simulink model "snap2_f_200msps_64i_4096c"  (R2019a)
settings: Solver=VariableStepDiscrete  StartTime=0.0  StopTime=10.0  RelTol=1e-3
undefined symbols (not defined in the file or in its folder): datetime, posixtime
libraries: xbsIndex_r4 x21354, casper_library_misc x297, casper_library_delays x19, xps_library x14, casper_library_sources x4
(part 9 of 217)

== system snap2_f_200msps_64i_4096c/autocorr/0 ==
  note: new_acc should precede data by a cycle
  note: acc length in spectra
  note: clock after sync counter goes to 1.
      |
      | Equality test goes high N spectra clock after sync. I.e., goes high with the last sample of the last spectra
  note: starts on 1
  sync : Inport
  din : Inport  Port=2
  rst : Inport  Port=3
  acc_len : Inport  Port=4
  trig : Inport  Port=5
  Convert{,1..7} (8 alike) : xbsIndex_r4/Convert  gui_display_data_type=Floating-point  arith_type=Floating-point  n_bits=16  bin_pt=14  float_type=Single  exp_bits=8  fraction_bits=24  quantization=Truncate  overflow=Wrap  en=off  latency=4  pipeline=on  dbl_ovrd=off  block_type=convert
  Counter : xbsIndex_r4/Counter  cnt_type=Free Running  cnt_to=Inf  operation=Up  start_count=1  cnt_by_val=1  arith_type=Unsigned  n_bits=30  bin_pt=0  load_pin=off  rst=on  en=off  explicit_period=on  period=1  use_behavioral_HDL=off  implementation=Fabric  dbl_ovrd=off  block_type=counter
  Delay : xbsIndex_r4/Delay  rst=off  infoeditControl=Selection of Reset will increase slice count due to use of real FFs and instead of SRLs  en=off  latency=1  reg_retiming=off  dbl_ovrd=off  block_type=delay
  Delay{1..16} (16 alike) : xbsIndex_r4/Delay  rst=off  infoeditControl=Selection of Reset will increase slice count due to use of real FFs and instead of SRLs  en=off  latency=4  reg_retiming=off  dbl_ovrd=off  block_type=delay
  Delay{17..32} (16 alike) : xbsIndex_r4/Delay  rst=off  infoeditControl=Selection of Reset will increase slice count due to use of real FFs and instead of SRLs  en=off  latency=1  reg_retiming=on  dbl_ovrd=off  block_type=delay
  Logical : xbsIndex_r4/Logical  logical_function=OR  inputs=2  en=off  latency=0  precision=Full  arith_type=Unsigned  n_bits=16  bin_pt=0  align_bp=on  dbl_ovrd=off  block_type=logical
  Logical{1..9} (9 alike) : xbsIndex_r4/Logical  logical_function=AND  inputs=2  en=off  latency=0  precision=Full  arith_type=Unsigned  n_bits=16  bin_pt=0  align_bp=on  dbl_ovrd=off  block_type=logical
  Register1 : xbsIndex_r4/Register  init=0  rst=on  en=on  dbl_ovrd=off  block_type=register
  Reinterpret{,1..7} (8 alike) : xbsIndex_r4/Reinterpret  force_arith_type=on  arith_type=Unsigned  force_bin_pt=on  bin_pt=0  block_type=reinterpret
  Relational : xbsIndex_r4/Relational  mode=a=b  op_type=Bool  en=off  latency=0  dbl_ovrd=off  block_type=relational
  Slice : xbsIndex_r4/Slice  nbits=30-nchan_bits-npol_bits  boolean_output=off  mode=Lower Bit Location + Width  bit1=0  base1=MSB of Input  bit0=nchan_bits + npol_bits  base0=LSB of Input  dbl_ovrd=off  block_type=slice
  bus_expand : Subsystem  AncestorBlock=casper_library_flow_control/bus_expand  mask(bus_expand){mode=divisions of equal size, outputNum=8, outputWidth=36, outputBinaryPt=0, outputArithmeticType=0, show_format=off, outputToWorkspace=off, variablePrefix=out, outputToModelAsWell=on}
      mask prompts: outputNum "Number of outputs:"; outputWidth "Output width:"; outputBinaryPt "Output binary point position:"; outputArithmeticType "Output arithmetic type (ufix=0, fix=1, bool=2):"; show_format "Print format string?"; outputToWorkspace "Output to workspace?"; variablePrefix "Variable name prefix:"; outputToModelAsWell "Output to model as well?"
      mask help:
      | Expands a 'bus' made using a bus_create or Xilinx
      | concat block.
      | The input will be divided into the specified number
      | of outputs with the specified arithmetic types.
      | Divisions are made from most significant bit.
      mask init: same as snap2_f_200msps_64i_4096c/autocorr/bus_expand
      settings: AttributesFormatString=8 outputs
      mask TypeOptions mode: divisions of equal size | divisions of arbitrary size
      mask Callback mode: bus_expand_callback();
      mask Callback outputWidth: bus_expand_callback();
      mask Callback outputToWorkspace: bus_expand_callback();
  dout0 : Subsystem
  dout1 : Subsystem
  dout2 : Subsystem
  dout3 : Subsystem
  dout4 : Subsystem
  dout5 : Subsystem
  dout6 : Subsystem
  dout7 : Subsystem
  edge_detect{,1..2,4} (4 alike) : casper_library_misc/edge_detect  edge=Rising  polarity=Active High  x_in=[0 0.08 0.08 0.16 0.16 0.24 0.24 0.32 0.32 0.4]  y_in="[-1 -1  1  1  1  1  1  1  1  1]"  x_out=[0.6 0.68 0.68 0.76 0.76 0.84 0.84 0.92 0.92 1]  y_out="[-1 -1  1  1 -1 -1 -1 -1 -1 -1]"
  edge_detect3 : Subsystem  AncestorBlock=casper_library_misc/edge_detect  mask(edge_detect){edge=Falling, polarity=Active High, x_in=[0 0.08 0.08 0.16 0.16 0.24 0.24 0.32 0.32 0.4], y_in=[-1 -1  1  1  1  1  1  1  1  1], x_out=[0.6 0.68 0.68 0.76 0.76 0.84 0.84 0.92 0.92 1], y_out=[-1 -1  1  1 -1 -1 -1 -1 -1 -1]}
      mask prompts: edge "Edge Type"; polarity "Output Polarity"; x_in "Input X Positions"; y_in "Input Y Positions"; x_out "Output X Positions"; y_out "Output Y Positions"
      mask help: Output is active for one-cycle after each edge of the specified type (i.e. rising, falling or both).
      mask init: same as snap2_f_200msps_64i_4096c/cosmic_ray/edge_detect
      settings: AttributesFormatString=|
      | falling edges
      | active high
      mask Help: Output is active for one-cycle after each edge of the specified type (i.e. rising, falling, or both).  Latency is zero.
      mask TypeOptions edge: Rising | Falling | Both
      mask TypeOptions polarity: Active High | Active Low
      mask Display:
      | plot(x_in_num,0.5+y_in_num*0.2);
      | plot(x_out_num,0.5+y_out_num*0.2);
  en_reg : xbsIndex_r4/Register  init=0  rst=on  en=on  dbl_ovrd=off  block_type=register
  power_dsp48e{,1..7} (8 alike) : casper_library_misc/power_dsp48e  bitwidth=18
      settings: SourceProductName=CASPER DSP Blockset
  simple_bram_vacc0 : Subsystem  AncestorBlock=casper_library_accumulators/simple_bram_vacc  mask(simple_bram_vacc){vec_len=2^(nchan_bits + npol_bits), arith_type=Signed, n_bits=64, bin_pt=17*2}
      mask prompts: vec_len "Vector length:"; arith_type "Output type:"; n_bits "Bit width (output):"; bin_pt "Binary point (output):"
      mask help: This simple vector accumulator is based on a shift register. It outputs its previous accumulated vector after a new_acc pulse is received.
      mask init:
      | simple_bram_vacc_init(gcb, ...
      |     'vec_len', vec_len, ...
      |     'arith_type', arith_type, ...
      |     'n_bits', n_bits, ...
      |     'bin_pt', bin_pt);
      mask TypeOptions arith_type: Signed | Unsigned
  simple_bram_vacc1 : Subsystem  AncestorBlock=casper_library_accumulators/simple_bram_vacc  mask(simple_bram_vacc){vec_len=2^(nchan_bits + npol_bits), arith_type=Signed, n_bits=64, bin_pt=17*2}
      mask prompts: vec_len "Vector length:"; arith_type "Output type:"; n_bits "Bit width (output):"; bin_pt "Binary point (output):"
      mask help: This simple vector accumulator is based on a shift register. It outputs its previous accumulated vector after a new_acc pulse is received.
      mask init:
      | simple_bram_vacc_init(gcb, ...
      |     'vec_len', vec_len, ...
      |     'arith_type', arith_type, ...
      |     'n_bits', n_bits, ...
      |     'bin_pt', bin_pt);
      mask TypeOptions arith_type: Signed | Unsigned
  simple_bram_vacc2 : Subsystem  AncestorBlock=casper_library_accumulators/simple_bram_vacc  mask(simple_bram_vacc){vec_len=2^(nchan_bits + npol_bits), arith_type=Signed, n_bits=64, bin_pt=17*2}
      mask prompts: vec_len "Vector length:"; arith_type "Output type:"; n_bits "Bit width (output):"; bin_pt "Binary point (output):"
      mask help: This simple vector accumulator is based on a shift register. It outputs its previous accumulated vector after a new_acc pulse is received.
      mask init:
      | simple_bram_vacc_init(gcb, ...
      |     'vec_len', vec_len, ...
      |     'arith_type', arith_type, ...
      |     'n_bits', n_bits, ...
      |     'bin_pt', bin_pt);
      mask TypeOptions arith_type: Signed | Unsigned
  simple_bram_vacc3 : Subsystem  AncestorBlock=casper_library_accumulators/simple_bram_vacc  mask(simple_bram_vacc){vec_len=2^(nchan_bits + npol_bits), arith_type=Signed, n_bits=64, bin_pt=17*2}
      mask prompts: vec_len "Vector length:"; arith_type "Output type:"; n_bits "Bit width (output):"; bin_pt "Binary point (output):"
      mask help: This simple vector accumulator is based on a shift register. It outputs its previous accumulated vector after a new_acc pulse is received.
      mask init:
      | simple_bram_vacc_init(gcb, ...
      |     'vec_len', vec_len, ...
      |     'arith_type', arith_type, ...
      |     'n_bits', n_bits, ...
      |     'bin_pt', bin_pt);
      mask TypeOptions arith_type: Signed | Unsigned
  simple_bram_vacc4 : Subsystem  AncestorBlock=casper_library_accumulators/simple_bram_vacc  mask(simple_bram_vacc){vec_len=2^(nchan_bits + npol_bits), arith_type=Signed, n_bits=64, bin_pt=17*2}
      mask prompts: vec_len "Vector length:"; arith_type "Output type:"; n_bits "Bit width (output):"; bin_pt "Binary point (output):"
      mask help: This simple vector accumulator is based on a shift register. It outputs its previous accumulated vector after a new_acc pulse is received.
      mask init:
      | simple_bram_vacc_init(gcb, ...
      |     'vec_len', vec_len, ...
      |     'arith_type', arith_type, ...
      |     'n_bits', n_bits, ...
      |     'bin_pt', bin_pt);
      mask TypeOptions arith_type: Signed | Unsigned
  simple_bram_vacc5 : Subsystem  AncestorBlock=casper_library_accumulators/simple_bram_vacc  mask(simple_bram_vacc){vec_len=2^(nchan_bits + npol_bits), arith_type=Signed, n_bits=64, bin_pt=17*2}
      mask prompts: vec_len "Vector length:"; arith_type "Output type:"; n_bits "Bit width (output):"; bin_pt "Binary point (output):"
      mask help: This simple vector accumulator is based on a shift register. It outputs its previous accumulated vector after a new_acc pulse is received.
      mask init:
      | simple_bram_vacc_init(gcb, ...
      |     'vec_len', vec_len, ...
      |     'arith_type', arith_type, ...
      |     'n_bits', n_bits, ...
      |     'bin_pt', bin_pt);
      mask TypeOptions arith_type: Signed | Unsigned
  simple_bram_vacc6 : Subsystem  AncestorBlock=casper_library_accumulators/simple_bram_vacc  mask(simple_bram_vacc){vec_len=2^(nchan_bits + npol_bits), arith_type=Signed, n_bits=64, bin_pt=17*2}
      mask prompts: vec_len "Vector length:"; arith_type "Output type:"; n_bits "Bit width (output):"; bin_pt "Binary point (output):"
      mask help: This simple vector accumulator is based on a shift register. It outputs its previous accumulated vector after a new_acc pulse is received.
      mask init:
      | simple_bram_vacc_init(gcb, ...
      |     'vec_len', vec_len, ...
      |     'arith_type', arith_type, ...
      |     'n_bits', n_bits, ...
      |     'bin_pt', bin_pt);
      mask TypeOptions arith_type: Signed | Unsigned
  simple_bram_vacc7 : Subsystem  AncestorBlock=casper_library_accumulators/simple_bram_vacc  mask(simple_bram_vacc){vec_len=2^(nchan_bits + npol_bits), arith_type=Signed, n_bits=64, bin_pt=17*2}
      mask prompts: vec_len "Vector length:"; arith_type "Output type:"; n_bits "Bit width (output):"; bin_pt "Binary point (output):"
      mask help: This simple vector accumulator is based on a shift register. It outputs its previous accumulated vector after a new_acc pulse is received.
      mask init:
      | simple_bram_vacc_init(gcb, ...
      |     'vec_len', vec_len, ...
      |     'arith_type', arith_type, ...
      |     'n_bits', n_bits, ...
      |     'bin_pt', bin_pt);
      mask TypeOptions arith_type: Signed | Unsigned
  trig_reg : xbsIndex_r4/Register  init=0  rst=on  en=on  dbl_ovrd=off  block_type=register
  new_acc : Outport
  wires:
  trig/1 -> edge_detect2/1
  Delay32/1 -> Logical9/1
  Delay31/1 -> Logical8/1
  Delay30/1 -> Logical7/1
  Delay29/1 -> Logical6/1
  Delay28/1 -> Logical5/1
  Delay27/1 -> Logical4/1
  Delay26/1 -> Logical3/1
  Delay14/1 -> Delay30/1
  Delay13/1 -> Delay29/1
  Delay12/1 -> Delay28/1
  Delay11/1 -> Delay27/1
  Delay10/1 -> Delay26/1
  Delay25/1 -> Logical1/1
  Delay15/1 -> Delay31/1
  Delay16/1 -> Delay32/1
  Logical9/1 -> dout7/2(vld)
  Logical8/1 -> dout6/2(vld)
  Logical7/1 -> dout5/2(vld)
  Logical6/1 -> dout4/2(vld)
  Logical5/1 -> dout3/2(vld)
  [enable_write] -> Logical9/2
  [enable_write] -> Logical8/2
  [enable_write] -> Logical7/2
  [enable_write] -> Logical6/2
  [enable_write] -> Logical5/2
  [enable_write] -> Logical4/2
  Logical4/1 -> dout2/2(vld)
  Logical3/1 -> dout1/2(vld)
  [enable_write] -> Logical3/2
  [enable_write] -> Logical1/2
  en_reg/1 -> edge_detect4/1, [enable_write]
  Delay24/1 -> dout7/1(din)
  Delay23/1 -> dout6/1(din)
  Delay22/1 -> dout5/1(din)
  Delay21/1 -> dout4/1(din)
  Delay20/1 -> dout3/1(din)
  Delay19/1 -> dout2/1(din)
  Delay18/1 -> dout1/1(din)
  Delay17/1 -> dout0/1(din)
  Logical1/1 -> dout0/2(vld)
  edge_detect4/1 -> trig_reg/2
  edge_detect3/1(out) -> en_reg/2
  edge_detect/1 -> en_reg/3
  edge_detect2/1 -> trig_reg/1, trig_reg/3
  trig_reg/1 -> en_reg/1
  sync/1 -> Register1/2, Logical2/2
  Register1/1 -> Logical2/1
  rst/1 -> Register1/3, Register1/1
  edge_detect1/1 -> Logical/1, new_acc/1, [new_acc]
  Logical/1 -> Counter/1
  Counter/1 -> Slice/1
  bus_expand/1(msb_out8) -> power_dsp48e/1
  bus_expand/2(out7) -> power_dsp48e1/1
  bus_expand/3(out6) -> power_dsp48e2/1
  bus_expand/4(out5) -> power_dsp48e3/1
  bus_expand/5(out4) -> power_dsp48e4/1
  bus_expand/6(out3) -> power_dsp48e5/1
  bus_expand/7(out2) -> power_dsp48e6/1
  bus_expand/8(lsb_out1) -> power_dsp48e7/1
  [new_acc] -> Delay8/1
  [new_acc] -> Delay1/1
  [new_acc] -> Delay3/1
  [new_acc] -> Delay4/1
  [new_acc] -> Delay5/1
  [new_acc] -> Delay6/1
  [new_acc] -> Delay7/1
  [new_acc] -> Delay9/1
  power_dsp48e/1 -> simple_bram_vacc0/2(din)
  power_dsp48e1/1 -> simple_bram_vacc2/2(din)
  power_dsp48e2/1 -> simple_bram_vacc1/2(din)
  power_dsp48e3/1 -> simple_bram_vacc3/2(din)
  power_dsp48e4/1 -> simple_bram_vacc4/2(din)
  power_dsp48e5/1 -> simple_bram_vacc6/2(din)
  power_dsp48e6/1 -> simple_bram_vacc5/2(din)
  power_dsp48e7/1 -> simple_bram_vacc7/2(din)
  din/1 -> bus_expand/1(bus_in)
  simple_bram_vacc0/1(dout) -> Convert/1
  simple_bram_vacc0/2(valid) -> Delay2/1
  simple_bram_vacc2/2(valid) -> Delay10/1
  simple_bram_vacc1/2(valid) -> Delay11/1
  simple_bram_vacc3/2(valid) -> Delay12/1
  simple_bram_vacc4/1(dout) -> Convert4/1
  simple_bram_vacc4/2(valid) -> Delay13/1
  simple_bram_vacc6/2(valid) -> Delay14/1
  simple_bram_vacc5/2(valid) -> Delay15/1
  simple_bram_vacc7/2(valid) -> Delay16/1
  Slice/1 -> Relational/1
  Relational/1 -> edge_detect1/1
  Logical2/1 -> Logical/2
  acc_len/1 -> Delay/1
  Delay9/1 -> simple_bram_vacc7/1(new_acc)
  Delay7/1 -> simple_bram_vacc5/1(new_acc)
  Delay6/1 -> simple_bram_vacc6/1(new_acc)
  Delay5/1 -> simple_bram_vacc4/1(new_acc)
  Delay4/1 -> simple_bram_vacc3/1(new_acc)
  Delay3/1 -> simple_bram_vacc1/1(new_acc)
  Delay1/1 -> simple_bram_vacc2/1(new_acc)
  Delay8/1 -> simple_bram_vacc0/1(new_acc)
  Reinterpret/1 -> Delay17/1
  simple_bram_vacc2/1(dout) -> Convert1/1
  simple_bram_vacc1/1(dout) -> Convert2/1
  simple_bram_vacc3/1(dout) -> Convert3/1
  Convert4/1 -> Reinterpret4/1
  Convert5/1 -> Reinterpret5/1
  simple_bram_vacc5/1(dout) -> Convert6/1
  simple_bram_vacc7/1(dout) -> Convert7/1
  Delay/1 -> Relational/2
  Convert/1 -> Reinterpret/1
  Delay2/1 -> edge_detect/1, Delay25/1, edge_detect3/1(in)
  Convert1/1 -> Reinterpret1/1
  Convert2/1 -> Reinterpret2/1
  Convert3/1 -> Reinterpret3/1
  simple_bram_vacc6/1(dout) -> Convert5/1
  Convert6/1 -> Reinterpret6/1
  Convert7/1 -> Reinterpret7/1
  Reinterpret1/1 -> Delay18/1
  Reinterpret2/1 -> Delay19/1
  Reinterpret3/1 -> Delay20/1
  Reinterpret4/1 -> Delay21/1
  Reinterpret5/1 -> Delay22/1
  Reinterpret6/1 -> Delay23/1
  Reinterpret7/1 -> Delay24/1

== system snap2_f_200msps_64i_4096c/autocorr/1 ==
  note: starts on 1
  note: clock after sync counter goes to 1.
      |
      | Equality test goes high N spectra clock after sync. I.e., goes high with the last sample of the last spectra
  note: acc length in spectra
  note: new_acc should precede data by a cycle
  sync : Inport
  din : Inport  Port=2
  rst : Inport  Port=3
  acc_len : Inport  Port=4
  trig : Inport  Port=5
  Convert{,1..7} (8 alike) : xbsIndex_r4/Convert  gui_display_data_type=Floating-point  arith_type=Floating-point  n_bits=16  bin_pt=14  float_type=Single  exp_bits=8  fraction_bits=24  quantization=Truncate  overflow=Wrap  en=off  latency=4  pipeline=on  dbl_ovrd=off  block_type=convert
  Counter : xbsIndex_r4/Counter  cnt_type=Free Running  cnt_to=Inf  operation=Up  start_count=1  cnt_by_val=1  arith_type=Unsigned  n_bits=30  bin_pt=0  load_pin=off  rst=on  en=off  explicit_period=on  period=1  use_behavioral_HDL=off  implementation=Fabric  dbl_ovrd=off  block_type=counter
  Delay : xbsIndex_r4/Delay  rst=off  infoeditControl=Selection of Reset will increase slice count due to use of real FFs and instead of SRLs  en=off  latency=1  reg_retiming=off  dbl_ovrd=off  block_type=delay
  Delay{1..16} (16 alike) : xbsIndex_r4/Delay  rst=off  infoeditControl=Selection of Reset will increase slice count due to use of real FFs and instead of SRLs  en=off  latency=4  reg_retiming=off  dbl_ovrd=off  block_type=delay
  Delay{17..32} (16 alike) : xbsIndex_r4/Delay  rst=off  infoeditControl=Selection of Reset will increase slice count due to use of real FFs and instead of SRLs  en=off  latency=1  reg_retiming=on  dbl_ovrd=off  block_type=delay
  Logical : xbsIndex_r4/Logical  logical_function=OR  inputs=2  en=off  latency=0  precision=Full  arith_type=Unsigned  n_bits=16  bin_pt=0  align_bp=on  dbl_ovrd=off  block_type=logical
  Logical{1..9} (9 alike) : xbsIndex_r4/Logical  logical_function=AND  inputs=2  en=off  latency=0  precision=Full  arith_type=Unsigned  n_bits=16  bin_pt=0  align_bp=on  dbl_ovrd=off  block_type=logical
  Register1 : xbsIndex_r4/Register  init=0  rst=on  en=on  dbl_ovrd=off  block_type=register
  Reinterpret{,1..7} (8 alike) : xbsIndex_r4/Reinterpret  force_arith_type=on  arith_type=Unsigned  force_bin_pt=on  bin_pt=0  block_type=reinterpret
  Relational : xbsIndex_r4/Relational  mode=a=b  op_type=Bool  en=off  latency=0  dbl_ovrd=off  block_type=relational
  Slice : xbsIndex_r4/Slice  nbits=30-nchan_bits-npol_bits  boolean_output=off  mode=Lower Bit Location + Width  bit1=0  base1=MSB of Input  bit0=nchan_bits + npol_bits  base0=LSB of Input  dbl_ovrd=off  block_type=slice
  bus_expand : Subsystem  AncestorBlock=casper_library_flow_control/bus_expand  mask(bus_expand){mode=divisions of equal size, outputNum=8, outputWidth=36, outputBinaryPt=0, outputArithmeticType=0, show_format=off, outputToWorkspace=off, variablePrefix=out, outputToModelAsWell=on}
      mask prompts: outputNum "Number of outputs:"; outputWidth "Output width:"; outputBinaryPt "Output binary point position:"; outputArithmeticType "Output arithmetic type (ufix=0, fix=1, bool=2):"; show_format "Print format string?"; outputToWorkspace "Output to workspace?"; variablePrefix "Variable name prefix:"; outputToModelAsWell "Output to model as well?"
      mask help:
      | Expands a 'bus' made using a bus_create or Xilinx
      | concat block.
      | The input will be divided into the specified number
      | of outputs with the specified arithmetic types.
      | Divisions are made from most significant bit.
      mask init: same as snap2_f_200msps_64i_4096c/autocorr/bus_expand
      settings: AttributesFormatString=8 outputs
      mask TypeOptions mode: divisions of equal size | divisions of arbitrary size
      mask Callback mode: bus_expand_callback();
      mask Callback outputWidth: bus_expand_callback();
      mask Callback outputToWorkspace: bus_expand_callback();
  dout0 : Subsystem
  dout1 : Subsystem
  dout2 : Subsystem
  dout3 : Subsystem
  dout4 : Subsystem
  dout5 : Subsystem
  dout6 : Subsystem
  dout7 : Subsystem
  edge_detect{,1..2,4} (4 alike) : casper_library_misc/edge_detect  edge=Rising  polarity=Active High  x_in=[0 0.08 0.08 0.16 0.16 0.24 0.24 0.32 0.32 0.4]  y_in="[-1 -1  1  1  1  1  1  1  1  1]"  x_out=[0.6 0.68 0.68 0.76 0.76 0.84 0.84 0.92 0.92 1]  y_out="[-1 -1  1  1 -1 -1 -1 -1 -1 -1]"
  edge_detect3 : Subsystem  AncestorBlock=casper_library_misc/edge_detect  mask(edge_detect){edge=Falling, polarity=Active High, x_in=[0 0.08 0.08 0.16 0.16 0.24 0.24 0.32 0.32 0.4], y_in=[-1 -1  1  1  1  1  1  1  1  1], x_out=[0.6 0.68 0.68 0.76 0.76 0.84 0.84 0.92 0.92 1], y_out=[-1 -1  1  1 -1 -1 -1 -1 -1 -1]}
      mask prompts: edge "Edge Type"; polarity "Output Polarity"; x_in "Input X Positions"; y_in "Input Y Positions"; x_out "Output X Positions"; y_out "Output Y Positions"
      mask help: Output is active for one-cycle after each edge of the specified type (i.e. rising, falling or both).
      mask init: same as snap2_f_200msps_64i_4096c/cosmic_ray/edge_detect
      settings: AttributesFormatString=|
      | falling edges
      | active high
      mask Help: Output is active for one-cycle after each edge of the specified type (i.e. rising, falling, or both).  Latency is zero.
      mask TypeOptions edge: Rising | Falling | Both
      mask TypeOptions polarity: Active High | Active Low
      mask Display:
      | plot(x_in_num,0.5+y_in_num*0.2);
      | plot(x_out_num,0.5+y_out_num*0.2);
  en_reg : xbsIndex_r4/Register  init=0  rst=on  en=on  dbl_ovrd=off  block_type=register
  power_dsp48e{,1..7} (8 alike) : casper_library_misc/power_dsp48e  bitwidth=18
      settings: SourceProductName=CASPER DSP Blockset
  simple_bram_vacc0 : Subsystem  AncestorBlock=casper_library_accumulators/simple_bram_vacc  mask(simple_bram_vacc){vec_len=2^(nchan_bits + npol_bits), arith_type=Signed, n_bits=64, bin_pt=17*2}
      mask prompts: vec_len "Vector length:"; arith_type "Output type:"; n_bits "Bit width (output):"; bin_pt "Binary point (output):"
      mask help: This simple vector accumulator is based on a shift register. It outputs its previous accumulated vector after a new_acc pulse is received.
      mask init:
      | simple_bram_vacc_init(gcb, ...
      |     'vec_len', vec_len, ...
      |     'arith_type', arith_type, ...
      |     'n_bits', n_bits, ...
      |     'bin_pt', bin_pt);
      mask TypeOptions arith_type: Signed | Unsigned
  simple_bram_vacc1 : Subsystem  AncestorBlock=casper_library_accumulators/simple_bram_vacc  mask(simple_bram_vacc){vec_len=2^(nchan_bits + npol_bits), arith_type=Signed, n_bits=64, bin_pt=17*2}
      mask prompts: vec_len "Vector length:"; arith_type "Output type:"; n_bits "Bit width (output):"; bin_pt "Binary point (output):"
      mask help: This simple vector accumulator is based on a shift register. It outputs its previous accumulated vector after a new_acc pulse is received.
      mask init:
      | simple_bram_vacc_init(gcb, ...
      |     'vec_len', vec_len, ...
      |     'arith_type', arith_type, ...
      |     'n_bits', n_bits, ...
      |     'bin_pt', bin_pt);
      mask TypeOptions arith_type: Signed | Unsigned
  simple_bram_vacc2 : Subsystem  AncestorBlock=casper_library_accumulators/simple_bram_vacc  mask(simple_bram_vacc){vec_len=2^(nchan_bits + npol_bits), arith_type=Signed, n_bits=64, bin_pt=17*2}
      mask prompts: vec_len "Vector length:"; arith_type "Output type:"; n_bits "Bit width (output):"; bin_pt "Binary point (output):"
      mask help: This simple vector accumulator is based on a shift register. It outputs its previous accumulated vector after a new_acc pulse is received.
      mask init:
      | simple_bram_vacc_init(gcb, ...
      |     'vec_len', vec_len, ...
      |     'arith_type', arith_type, ...
      |     'n_bits', n_bits, ...
      |     'bin_pt', bin_pt);
      mask TypeOptions arith_type: Signed | Unsigned
  simple_bram_vacc3 : Subsystem  AncestorBlock=casper_library_accumulators/simple_bram_vacc  mask(simple_bram_vacc){vec_len=2^(nchan_bits + npol_bits), arith_type=Signed, n_bits=64, bin_pt=17*2}
      mask prompts: vec_len "Vector length:"; arith_type "Output type:"; n_bits "Bit width (output):"; bin_pt "Binary point (output):"
      mask help: This simple vector accumulator is based on a shift register. It outputs its previous accumulated vector after a new_acc pulse is received.
      mask init:
      | simple_bram_vacc_init(gcb, ...
      |     'vec_len', vec_len, ...
      |     'arith_type', arith_type, ...
      |     'n_bits', n_bits, ...
      |     'bin_pt', bin_pt);
      mask TypeOptions arith_type: Signed | Unsigned
  simple_bram_vacc4 : Subsystem  AncestorBlock=casper_library_accumulators/simple_bram_vacc  mask(simple_bram_vacc){vec_len=2^(nchan_bits + npol_bits), arith_type=Signed, n_bits=64, bin_pt=17*2}
      mask prompts: vec_len "Vector length:"; arith_type "Output type:"; n_bits "Bit width (output):"; bin_pt "Binary point (output):"
      mask help: This simple vector accumulator is based on a shift register. It outputs its previous accumulated vector after a new_acc pulse is received.
      mask init:
      | simple_bram_vacc_init(gcb, ...
      |     'vec_len', vec_len, ...
      |     'arith_type', arith_type, ...
      |     'n_bits', n_bits, ...
      |     'bin_pt', bin_pt);
      mask TypeOptions arith_type: Signed | Unsigned
  simple_bram_vacc5 : Subsystem  AncestorBlock=casper_library_accumulators/simple_bram_vacc  mask(simple_bram_vacc){vec_len=2^(nchan_bits + npol_bits), arith_type=Signed, n_bits=64, bin_pt=17*2}
      mask prompts: vec_len "Vector length:"; arith_type "Output type:"; n_bits "Bit width (output):"; bin_pt "Binary point (output):"
      mask help: This simple vector accumulator is based on a shift register. It outputs its previous accumulated vector after a new_acc pulse is received.
      mask init:
      | simple_bram_vacc_init(gcb, ...
      |     'vec_len', vec_len, ...
      |     'arith_type', arith_type, ...
      |     'n_bits', n_bits, ...
      |     'bin_pt', bin_pt);
      mask TypeOptions arith_type: Signed | Unsigned
  simple_bram_vacc6 : Subsystem  AncestorBlock=casper_library_accumulators/simple_bram_vacc  mask(simple_bram_vacc){vec_len=2^(nchan_bits + npol_bits), arith_type=Signed, n_bits=64, bin_pt=17*2}
      mask prompts: vec_len "Vector length:"; arith_type "Output type:"; n_bits "Bit width (output):"; bin_pt "Binary point (output):"
      mask help: This simple vector accumulator is based on a shift register. It outputs its previous accumulated vector after a new_acc pulse is received.
      mask init:
      | simple_bram_vacc_init(gcb, ...
      |     'vec_len', vec_len, ...
      |     'arith_type', arith_type, ...
      |     'n_bits', n_bits, ...
      |     'bin_pt', bin_pt);
      mask TypeOptions arith_type: Signed | Unsigned
  simple_bram_vacc7 : Subsystem  AncestorBlock=casper_library_accumulators/simple_bram_vacc  mask(simple_bram_vacc){vec_len=2^(nchan_bits + npol_bits), arith_type=Signed, n_bits=64, bin_pt=17*2}
      mask prompts: vec_len "Vector length:"; arith_type "Output type:"; n_bits "Bit width (output):"; bin_pt "Binary point (output):"
      mask help: This simple vector accumulator is based on a shift register. It outputs its previous accumulated vector after a new_acc pulse is received.
      mask init:
      | simple_bram_vacc_init(gcb, ...
      |     'vec_len', vec_len, ...
      |     'arith_type', arith_type, ...
      |     'n_bits', n_bits, ...
      |     'bin_pt', bin_pt);
      mask TypeOptions arith_type: Signed | Unsigned
  trig_reg : xbsIndex_r4/Register  init=0  rst=on  en=on  dbl_ovrd=off  block_type=register
  new_acc : Outport
  wires:
  Reinterpret7/1 -> Delay24/1
  Reinterpret6/1 -> Delay23/1
  Reinterpret5/1 -> Delay22/1
  Reinterpret4/1 -> Delay21/1
  Reinterpret3/1 -> Delay20/1
  Reinterpret2/1 -> Delay19/1
  Reinterpret1/1 -> Delay18/1
  Convert7/1 -> Reinterpret7/1
  Convert6/1 -> Reinterpret6/1
  simple_bram_vacc6/1(dout) -> Convert5/1
  Convert3/1 -> Reinterpret3/1
  Convert2/1 -> Reinterpret2/1
  Convert1/1 -> Reinterpret1/1
  Delay2/1 -> edge_detect3/1(in), Delay25/1, edge_detect/1
  Convert/1 -> Reinterpret/1
  Delay/1 -> Relational/2
  simple_bram_vacc7/1(dout) -> Convert7/1
  simple_bram_vacc5/1(dout) -> Convert6/1
  Convert5/1 -> Reinterpret5/1
  Convert4/1 -> Reinterpret4/1
  simple_bram_vacc3/1(dout) -> Convert3/1
  simple_bram_vacc1/1(dout) -> Convert2/1
  simple_bram_vacc2/1(dout) -> Convert1/1
  Reinterpret/1 -> Delay17/1
  Delay8/1 -> simple_bram_vacc0/1(new_acc)
  Delay1/1 -> simple_bram_vacc2/1(new_acc)
  Delay3/1 -> simple_bram_vacc1/1(new_acc)
  Delay4/1 -> simple_bram_vacc3/1(new_acc)
  Delay5/1 -> simple_bram_vacc4/1(new_acc)
  Delay6/1 -> simple_bram_vacc6/1(new_acc)
  Delay7/1 -> simple_bram_vacc5/1(new_acc)
  Delay9/1 -> simple_bram_vacc7/1(new_acc)
  acc_len/1 -> Delay/1
  Logical2/1 -> Logical/2
  Relational/1 -> edge_detect1/1
  Slice/1 -> Relational/1
  simple_bram_vacc7/2(valid) -> Delay16/1
  simple_bram_vacc5/2(valid) -> Delay15/1
  simple_bram_vacc6/2(valid) -> Delay14/1
  simple_bram_vacc4/2(valid) -> Delay13/1
  simple_bram_vacc4/1(dout) -> Convert4/1
  simple_bram_vacc3/2(valid) -> Delay12/1
  simple_bram_vacc1/2(valid) -> Delay11/1
  simple_bram_vacc2/2(valid) -> Delay10/1
  simple_bram_vacc0/2(valid) -> Delay2/1
  simple_bram_vacc0/1(dout) -> Convert/1
  din/1 -> bus_expand/1(bus_in)
  power_dsp48e7/1 -> simple_bram_vacc7/2(din)
  power_dsp48e6/1 -> simple_bram_vacc5/2(din)
  power_dsp48e5/1 -> simple_bram_vacc6/2(din)
  power_dsp48e4/1 -> simple_bram_vacc4/2(din)
  power_dsp48e3/1 -> simple_bram_vacc3/2(din)
  power_dsp48e2/1 -> simple_bram_vacc1/2(din)
  power_dsp48e1/1 -> simple_bram_vacc2/2(din)
  power_dsp48e/1 -> simple_bram_vacc0/2(din)
  [new_acc] -> Delay9/1
  [new_acc] -> Delay7/1
  [new_acc] -> Delay6/1
  [new_acc] -> Delay5/1
  [new_acc] -> Delay4/1
  [new_acc] -> Delay3/1
  [new_acc] -> Delay1/1
  [new_acc] -> Delay8/1
  bus_expand/8(lsb_out1) -> power_dsp48e7/1
  bus_expand/7(out2) -> power_dsp48e6/1
  bus_expand/6(out3) -> power_dsp48e5/1
  bus_expand/5(out4) -> power_dsp48e4/1
  bus_expand/4(out5) -> power_dsp48e3/1
  bus_expand/3(out6) -> power_dsp48e2/1
  bus_expand/2(out7) -> power_dsp48e1/1
  bus_expand/1(msb_out8) -> power_dsp48e/1
  Counter/1 -> Slice/1
  Logical/1 -> Counter/1
  edge_detect1/1 -> [new_acc], new_acc/1, Logical/1
  rst/1 -> Register1/1, Register1/3
  Register1/1 -> Logical2/1
  sync/1 -> Logical2/2, Register1/2
  trig_reg/1 -> en_reg/1
  edge_detect2/1 -> trig_reg/3, trig_reg/1
  edge_detect/1 -> en_reg/3
  edge_detect3/1(out) -> en_reg/2
  edge_detect4/1 -> trig_reg/2
  Logical1/1 -> dout0/2(vld)
  Delay17/1 -> dout0/1(din)
  Delay18/1 -> dout1/1(din)
  Delay19/1 -> dout2/1(din)
  Delay20/1 -> dout3/1(din)
  Delay21/1 -> dout4/1(din)
  Delay22/1 -> dout5/1(din)
  Delay23/1 -> dout6/1(din)
  Delay24/1 -> dout7/1(din)
  en_reg/1 -> [enable_write], edge_detect4/1
  [enable_write] -> Logical1/2
  [enable_write] -> Logical3/2
  Logical3/1 -> dout1/2(vld)
  Logical4/1 -> dout2/2(vld)
  [enable_write] -> Logical4/2
  [enable_write] -> Logical5/2
  [enable_write] -> Logical6/2
  [enable_write] -> Logical7/2
  [enable_write] -> Logical8/2
  [enable_write] -> Logical9/2
  Logical5/1 -> dout3/2(vld)
  Logical6/1 -> dout4/2(vld)
  Logical7/1 -> dout5/2(vld)
  Logical8/1 -> dout6/2(vld)
  Logical9/1 -> dout7/2(vld)
  Delay16/1 -> Delay32/1
  Delay15/1 -> Delay31/1
  Delay25/1 -> Logical1/1
  Delay10/1 -> Delay26/1
  Delay11/1 -> Delay27/1
  Delay12/1 -> Delay28/1
  Delay13/1 -> Delay29/1
  Delay14/1 -> Delay30/1
  Delay26/1 -> Logical3/1
  Delay27/1 -> Logical4/1
  Delay28/1 -> Logical5/1
  Delay29/1 -> Logical6/1
  Delay30/1 -> Logical7/1
  Delay31/1 -> Logical8/1
  Delay32/1 -> Logical9/1
  trig/1 -> edge_detect2/1

== system snap2_f_200msps_64i_4096c/autocorr/2 ==
  note: new_acc should precede data by a cycle
  note: acc length in spectra
  note: clock after sync counter goes to 1.
      |
      | Equality test goes high N spectra clock after sync. I.e., goes high with the last sample of the last spectra
  note: starts on 1
  sync : Inport
  din : Inport  Port=2
  rst : Inport  Port=3
  acc_len : Inport  Port=4
  trig : Inport  Port=5
  Convert{,1..7} (8 alike) : xbsIndex_r4/Convert  gui_display_data_type=Floating-point  arith_type=Floating-point  n_bits=16  bin_pt=14  float_type=Single  exp_bits=8  fraction_bits=24  quantization=Truncate  overflow=Wrap  en=off  latency=4  pipeline=on  dbl_ovrd=off  block_type=convert
  Counter : xbsIndex_r4/Counter  cnt_type=Free Running  cnt_to=Inf  operation=Up  start_count=1  cnt_by_val=1  arith_type=Unsigned  n_bits=30  bin_pt=0  load_pin=off  rst=on  en=off  explicit_period=on  period=1  use_behavioral_HDL=off  implementation=Fabric  dbl_ovrd=off  block_type=counter
  Delay : xbsIndex_r4/Delay  rst=off  infoeditControl=Selection of Reset will increase slice count due to use of real FFs and instead of SRLs  en=off  latency=1  reg_retiming=off  dbl_ovrd=off  block_type=delay
  Delay{1..16} (16 alike) : xbsIndex_r4/Delay  rst=off  infoeditControl=Selection of Reset will increase slice count due to use of real FFs and instead of SRLs  en=off  latency=4  reg_retiming=off  dbl_ovrd=off  block_type=delay
  Delay{17..32} (16 alike) : xbsIndex_r4/Delay  rst=off  infoeditControl=Selection of Reset will increase slice count due to use of real FFs and instead of SRLs  en=off  latency=1  reg_retiming=on  dbl_ovrd=off  block_type=delay
  Logical : xbsIndex_r4/Logical  logical_function=OR  inputs=2  en=off  latency=0  precision=Full  arith_type=Unsigned  n_bits=16  bin_pt=0  align_bp=on  dbl_ovrd=off  block_type=logical
  Logical{1..9} (9 alike) : xbsIndex_r4/Logical  logical_function=AND  inputs=2  en=off  latency=0  precision=Full  arith_type=Unsigned  n_bits=16  bin_pt=0  align_bp=on  dbl_ovrd=off  block_type=logical
  Register1 : xbsIndex_r4/Register  init=0  rst=on  en=on  dbl_ovrd=off  block_type=register
  Reinterpret{,1..7} (8 alike) : xbsIndex_r4/Reinterpret  force_arith_type=on  arith_type=Unsigned  force_bin_pt=on  bin_pt=0  block_type=reinterpret
  Relational : xbsIndex_r4/Relational  mode=a=b  op_type=Bool  en=off  latency=0  dbl_ovrd=off  block_type=relational
  Slice : xbsIndex_r4/Slice  nbits=30-nchan_bits-npol_bits  boolean_output=off  mode=Lower Bit Location + Width  bit1=0  base1=MSB of Input  bit0=nchan_bits + npol_bits  base0=LSB of Input  dbl_ovrd=off  block_type=slice
  bus_expand : Subsystem  AncestorBlock=casper_library_flow_control/bus_expand  mask(bus_expand){mode=divisions of equal size, outputNum=8, outputWidth=36, outputBinaryPt=0, outputArithmeticType=0, show_format=off, outputToWorkspace=off, variablePrefix=out, outputToModelAsWell=on}
      mask prompts: outputNum "Number of outputs:"; outputWidth "Output width:"; outputBinaryPt "Output binary point position:"; outputArithmeticType "Output arithmetic type (ufix=0, fix=1, bool=2):"; show_format "Print format string?"; outputToWorkspace "Output to workspace?"; variablePrefix "Variable name prefix:"; outputToModelAsWell "Output to model as well?"
      mask help:
      | Expands a 'bus' made using a bus_create or Xilinx
      | concat block.
      | The input will be divided into the specified number
      | of outputs with the specified arithmetic types.
      | Divisions are made from most significant bit.
      mask init: same as snap2_f_200msps_64i_4096c/autocorr/bus_expand
      settings: AttributesFormatString=8 outputs
      mask TypeOptions mode: divisions of equal size | divisions of arbitrary size
      mask Callback mode: bus_expand_callback();
      mask Callback outputWidth: bus_expand_callback();
      mask Callback outputToWorkspace: bus_expand_callback();
  dout0 : Subsystem
  dout1 : Subsystem
  dout2 : Subsystem
  dout3 : Subsystem
  dout4 : Subsystem
  dout5 : Subsystem
  dout6 : Subsystem
  dout7 : Subsystem
  edge_detect{,1..2,4} (4 alike) : casper_library_misc/edge_detect  edge=Rising  polarity=Active High  x_in=[0 0.08 0.08 0.16 0.16 0.24 0.24 0.32 0.32 0.4]  y_in="[-1 -1  1  1  1  1  1  1  1  1]"  x_out=[0.6 0.68 0.68 0.76 0.76 0.84 0.84 0.92 0.92 1]  y_out="[-1 -1  1  1 -1 -1 -1 -1 -1 -1]"
  edge_detect3 : Subsystem  AncestorBlock=casper_library_misc/edge_detect  mask(edge_detect){edge=Falling, polarity=Active High, x_in=[0 0.08 0.08 0.16 0.16 0.24 0.24 0.32 0.32 0.4], y_in=[-1 -1  1  1  1  1  1  1  1  1], x_out=[0.6 0.68 0.68 0.76 0.76 0.84 0.84 0.92 0.92 1], y_out=[-1 -1  1  1 -1 -1 -1 -1 -1 -1]}
      mask prompts: edge "Edge Type"; polarity "Output Polarity"; x_in "Input X Positions"; y_in "Input Y Positions"; x_out "Output X Positions"; y_out "Output Y Positions"
      mask help: Output is active for one-cycle after each edge of the specified type (i.e. rising, falling or both).
      mask init: same as snap2_f_200msps_64i_4096c/cosmic_ray/edge_detect
      settings: AttributesFormatString=|
      | falling edges
      | active high
      mask Help: Output is active for one-cycle after each edge of the specified type (i.e. rising, falling, or both).  Latency is zero.
      mask TypeOptions edge: Rising | Falling | Both
      mask TypeOptions polarity: Active High | Active Low
      mask Display:
      | plot(x_in_num,0.5+y_in_num*0.2);
      | plot(x_out_num,0.5+y_out_num*0.2);
  en_reg : xbsIndex_r4/Register  init=0  rst=on  en=on  dbl_ovrd=off  block_type=register
  power_dsp48e{,1..7} (8 alike) : casper_library_misc/power_dsp48e  bitwidth=18
      settings: SourceProductName=CASPER DSP Blockset
  simple_bram_vacc0 : Subsystem  AncestorBlock=casper_library_accumulators/simple_bram_vacc  mask(simple_bram_vacc){vec_len=2^(nchan_bits + npol_bits), arith_type=Signed, n_bits=64, bin_pt=17*2}
      mask prompts: vec_len "Vector length:"; arith_type "Output type:"; n_bits "Bit width (output):"; bin_pt "Binary point (output):"
      mask help: This simple vector accumulator is based on a shift register. It outputs its previous accumulated vector after a new_acc pulse is received.
      mask init:
      | simple_bram_vacc_init(gcb, ...
      |     'vec_len', vec_len, ...
      |     'arith_type', arith_type, ...
      |     'n_bits', n_bits, ...
      |     'bin_pt', bin_pt);
      mask TypeOptions arith_type: Signed | Unsigned
  simple_bram_vacc1 : Subsystem  AncestorBlock=casper_library_accumulators/simple_bram_vacc  mask(simple_bram_vacc){vec_len=2^(nchan_bits + npol_bits), arith_type=Signed, n_bits=64, bin_pt=17*2}
      mask prompts: vec_len "Vector length:"; arith_type "Output type:"; n_bits "Bit width (output):"; bin_pt "Binary point (output):"
      mask help: This simple vector accumulator is based on a shift register. It outputs its previous accumulated vector after a new_acc pulse is received.
      mask init:
      | simple_bram_vacc_init(gcb, ...
      |     'vec_len', vec_len, ...
      |     'arith_type', arith_type, ...
      |     'n_bits', n_bits, ...
      |     'bin_pt', bin_pt);
      mask TypeOptions arith_type: Signed | Unsigned
  simple_bram_vacc2 : Subsystem  AncestorBlock=casper_library_accumulators/simple_bram_vacc  mask(simple_bram_vacc){vec_len=2^(nchan_bits + npol_bits), arith_type=Signed, n_bits=64, bin_pt=17*2}
      mask prompts: vec_len "Vector length:"; arith_type "Output type:"; n_bits "Bit width (output):"; bin_pt "Binary point (output):"
      mask help: This simple vector accumulator is based on a shift register. It outputs its previous accumulated vector after a new_acc pulse is received.
      mask init:
      | simple_bram_vacc_init(gcb, ...
      |     'vec_len', vec_len, ...
      |     'arith_type', arith_type, ...
      |     'n_bits', n_bits, ...
      |     'bin_pt', bin_pt);
      mask TypeOptions arith_type: Signed | Unsigned
  simple_bram_vacc3 : Subsystem  AncestorBlock=casper_library_accumulators/simple_bram_vacc  mask(simple_bram_vacc){vec_len=2^(nchan_bits + npol_bits), arith_type=Signed, n_bits=64, bin_pt=17*2}
      mask prompts: vec_len "Vector length:"; arith_type "Output type:"; n_bits "Bit width (output):"; bin_pt "Binary point (output):"
      mask help: This simple vector accumulator is based on a shift register. It outputs its previous accumulated vector after a new_acc pulse is received.
      mask init:
      | simple_bram_vacc_init(gcb, ...
      |     'vec_len', vec_len, ...
      |     'arith_type', arith_type, ...
      |     'n_bits', n_bits, ...
      |     'bin_pt', bin_pt);
      mask TypeOptions arith_type: Signed | Unsigned
  simple_bram_vacc4 : Subsystem  AncestorBlock=casper_library_accumulators/simple_bram_vacc  mask(simple_bram_vacc){vec_len=2^(nchan_bits + npol_bits), arith_type=Signed, n_bits=64, bin_pt=17*2}
      mask prompts: vec_len "Vector length:"; arith_type "Output type:"; n_bits "Bit width (output):"; bin_pt "Binary point (output):"
      mask help: This simple vector accumulator is based on a shift register. It outputs its previous accumulated vector after a new_acc pulse is received.
      mask init:
      | simple_bram_vacc_init(gcb, ...
      |     'vec_len', vec_len, ...
      |     'arith_type', arith_type, ...
      |     'n_bits', n_bits, ...
      |     'bin_pt', bin_pt);
      mask TypeOptions arith_type: Signed | Unsigned
  simple_bram_vacc5 : Subsystem  AncestorBlock=casper_library_accumulators/simple_bram_vacc  mask(simple_bram_vacc){vec_len=2^(nchan_bits + npol_bits), arith_type=Signed, n_bits=64, bin_pt=17*2}
      mask prompts: vec_len "Vector length:"; arith_type "Output type:"; n_bits "Bit width (output):"; bin_pt "Binary point (output):"
      mask help: This simple vector accumulator is based on a shift register. It outputs its previous accumulated vector after a new_acc pulse is received.
      mask init:
      | simple_bram_vacc_init(gcb, ...
      |     'vec_len', vec_len, ...
      |     'arith_type', arith_type, ...
      |     'n_bits', n_bits, ...
      |     'bin_pt', bin_pt);
      mask TypeOptions arith_type: Signed | Unsigned
  simple_bram_vacc6 : Subsystem  AncestorBlock=casper_library_accumulators/simple_bram_vacc  mask(simple_bram_vacc){vec_len=2^(nchan_bits + npol_bits), arith_type=Signed, n_bits=64, bin_pt=17*2}
      mask prompts: vec_len "Vector length:"; arith_type "Output type:"; n_bits "Bit width (output):"; bin_pt "Binary point (output):"
      mask help: This simple vector accumulator is based on a shift register. It outputs its previous accumulated vector after a new_acc pulse is received.
      mask init:
      | simple_bram_vacc_init(gcb, ...
      |     'vec_len', vec_len, ...
      |     'arith_type', arith_type, ...
      |     'n_bits', n_bits, ...
      |     'bin_pt', bin_pt);
      mask TypeOptions arith_type: Signed | Unsigned
  simple_bram_vacc7 : Subsystem  AncestorBlock=casper_library_accumulators/simple_bram_vacc  mask(simple_bram_vacc){vec_len=2^(nchan_bits + npol_bits), arith_type=Signed, n_bits=64, bin_pt=17*2}
      mask prompts: vec_len "Vector length:"; arith_type "Output type:"; n_bits "Bit width (output):"; bin_pt "Binary point (output):"
      mask help: This simple vector accumulator is based on a shift register. It outputs its previous accumulated vector after a new_acc pulse is received.
      mask init:
      | simple_bram_vacc_init(gcb, ...
      |     'vec_len', vec_len, ...
      |     'arith_type', arith_type, ...
      |     'n_bits', n_bits, ...
      |     'bin_pt', bin_pt);
      mask TypeOptions arith_type: Signed | Unsigned
  trig_reg : xbsIndex_r4/Register  init=0  rst=on  en=on  dbl_ovrd=off  block_type=register
  new_acc : Outport
  wires:
  trig/1 -> edge_detect2/1
  Delay32/1 -> Logical9/1
  Delay31/1 -> Logical8/1
  Delay30/1 -> Logical7/1
  Delay29/1 -> Logical6/1
  Delay28/1 -> Logical5/1
  Delay27/1 -> Logical4/1
  Delay26/1 -> Logical3/1
  Delay14/1 -> Delay30/1
  Delay13/1 -> Delay29/1
  Delay12/1 -> Delay28/1
  Delay11/1 -> Delay27/1
  Delay10/1 -> Delay26/1
  Delay25/1 -> Logical1/1
  Delay15/1 -> Delay31/1
  Delay16/1 -> Delay32/1
  Logical9/1 -> dout7/2(vld)
  Logical8/1 -> dout6/2(vld)
  Logical7/1 -> dout5/2(vld)
  Logical6/1 -> dout4/2(vld)
  Logical5/1 -> dout3/2(vld)
  [enable_write] -> Logical9/2
  [enable_write] -> Logical8/2
  [enable_write] -> Logical7/2
  [enable_write] -> Logical6/2
  [enable_write] -> Logical5/2
  [enable_write] -> Logical4/2
  Logical4/1 -> dout2/2(vld)
  Logical3/1 -> dout1/2(vld)
  [enable_write] -> Logical3/2
  [enable_write] -> Logical1/2
  en_reg/1 -> edge_detect4/1, [enable_write]
  Delay24/1 -> dout7/1(din)
  Delay23/1 -> dout6/1(din)
  Delay22/1 -> dout5/1(din)
  Delay21/1 -> dout4/1(din)
  Delay20/1 -> dout3/1(din)
  Delay19/1 -> dout2/1(din)
  Delay18/1 -> dout1/1(din)
  Delay17/1 -> dout0/1(din)
  Logical1/1 -> dout0/2(vld)
  edge_detect4/1 -> trig_reg/2
  edge_detect3/1(out) -> en_reg/2
  edge_detect/1 -> en_reg/3
  edge_detect2/1 -> trig_reg/1, trig_reg/3
  trig_reg/1 -> en_reg/1
  sync/1 -> Register1/2, Logical2/2
  Register1/1 -> Logical2/1
  rst/1 -> Register1/3, Register1/1
  edge_detect1/1 -> Logical/1, new_acc/1, [new_acc]
  Logical/1 -> Counter/1
  Counter/1 -> Slice/1
  bus_expand/1(msb_out8) -> power_dsp48e/1
  bus_expand/2(out7) -> power_dsp48e1/1
  bus_expand/3(out6) -> power_dsp48e2/1
  bus_expand/4(out5) -> power_dsp48e3/1
  bus_expand/5(out4) -> power_dsp48e4/1
  bus_expand/6(out3) -> power_dsp48e5/1
  bus_expand/7(out2) -> power_dsp48e6/1
  bus_expand/8(lsb_out1) -> power_dsp48e7/1
  [new_acc] -> Delay8/1
  [new_acc] -> Delay1/1
  [new_acc] -> Delay3/1
  [new_acc] -> Delay4/1
  [new_acc] -> Delay5/1
  [new_acc] -> Delay6/1
  [new_acc] -> Delay7/1
  [new_acc] -> Delay9/1
  power_dsp48e/1 -> simple_bram_vacc0/2(din)
  power_dsp48e1/1 -> simple_bram_vacc2/2(din)
  power_dsp48e2/1 -> simple_bram_vacc1/2(din)
  power_dsp48e3/1 -> simple_bram_vacc3/2(din)
  power_dsp48e4/1 -> simple_bram_vacc4/2(din)
  power_dsp48e5/1 -> simple_bram_vacc6/2(din)
  power_dsp48e6/1 -> simple_bram_vacc5/2(din)
  power_dsp48e7/1 -> simple_bram_vacc7/2(din)
  din/1 -> bus_expand/1(bus_in)
  simple_bram_vacc0/1(dout) -> Convert/1
  simple_bram_vacc0/2(valid) -> Delay2/1
  simple_bram_vacc2/2(valid) -> Delay10/1
  simple_bram_vacc1/2(valid) -> Delay11/1
  simple_bram_vacc3/2(valid) -> Delay12/1
  simple_bram_vacc4/1(dout) -> Convert4/1
  simple_bram_vacc4/2(valid) -> Delay13/1
  simple_bram_vacc6/2(valid) -> Delay14/1
  simple_bram_vacc5/2(valid) -> Delay15/1
  simple_bram_vacc7/2(valid) -> Delay16/1
  Slice/1 -> Relational/1
  Relational/1 -> edge_detect1/1
  Logical2/1 -> Logical/2
  acc_len/1 -> Delay/1
  Delay9/1 -> simple_bram_vacc7/1(new_acc)
  Delay7/1 -> simple_bram_vacc5/1(new_acc)
  Delay6/1 -> simple_bram_vacc6/1(new_acc)
  Delay5/1 -> simple_bram_vacc4/1(new_acc)
  Delay4/1 -> simple_bram_vacc3/1(new_acc)
  Delay3/1 -> simple_bram_vacc1/1(new_acc)
  Delay1/1 -> simple_bram_vacc2/1(new_acc)
  Delay8/1 -> simple_bram_vacc0/1(new_acc)
  Reinterpret/1 -> Delay17/1
  simple_bram_vacc2/1(dout) -> Convert1/1
  simple_bram_vacc1/1(dout) -> Convert2/1
  simple_bram_vacc3/1(dout) -> Convert3/1
  Convert4/1 -> Reinterpret4/1
  Convert5/1 -> Reinterpret5/1
  simple_bram_vacc5/1(dout) -> Convert6/1
  simple_bram_vacc7/1(dout) -> Convert7/1
  Delay/1 -> Relational/2
  Convert/1 -> Reinterpret/1
  Delay2/1 -> edge_detect/1, Delay25/1, edge_detect3/1(in)
  Convert1/1 -> Reinterpret1/1
  Convert2/1 -> Reinterpret2/1
  Convert3/1 -> Reinterpret3/1
  simple_bram_vacc6/1(dout) -> Convert5/1
  Convert6/1 -> Reinterpret6/1
  Convert7/1 -> Reinterpret7/1
  Reinterpret1/1 -> Delay18/1
  Reinterpret2/1 -> Delay19/1
  Reinterpret3/1 -> Delay20/1
  Reinterpret4/1 -> Delay21/1
  Reinterpret5/1 -> Delay22/1
  Reinterpret6/1 -> Delay23/1
  Reinterpret7/1 -> Delay24/1
